simulink model "EST2"  (R2023b)
settings: Solver=FixedStepAuto  StartTime=0.0  StopTime=stopt  FixedStep=deltat  MaxStep=0.05  RelTol=1e-3
InitFcn:
  | clear all;
  | close all;
  | clc;
  | 
  | % add the data and script directories
  | addpath('data','scripts');
  | 
  | % load the constants (units)
  | constants;
  | 
  | % load the simulation parameters
  | preprocessing;
StopFcn:
  | postprocessing;
values from neighbouring files (symbols this model uses):
  aDemandTransport = aSupplyTransport    (= 0.97)    [preprocessing.m]
  aExtraction = 1- eta_extr    (= 0.1561)    [preprocessing.m]
  aSupplyTransport = 0.97    [preprocessing.m]
  bStorage = 0    [preprocessing.m]
  deltat = 5*unit("min")    [preprocessing.m]
  EStorageInitial = EStorageMax/2    (= 500000000000)    [preprocessing.m]
  EStorageMax = 1e12    (= 1000000000000)    [preprocessing.m]
  EStorageMin = EStorageMax/20    (= 50000000000)    [preprocessing.m]
  N_sphere = 35    [preprocessing.m]
  r_sph = 6.2    [preprocessing.m]
settings Model: Creator=joche  LastModifiedBy=20241276
settings DataIOCC: SaveFormat=Array  SaveOutput=off  ReturnWorkspaceOutputs=off
settings OptimizationCC: ReuseModelBlockBuffer=off
settings ModelReferenceCC: EnableRefExpFcnMdlSchedulingChecks=on

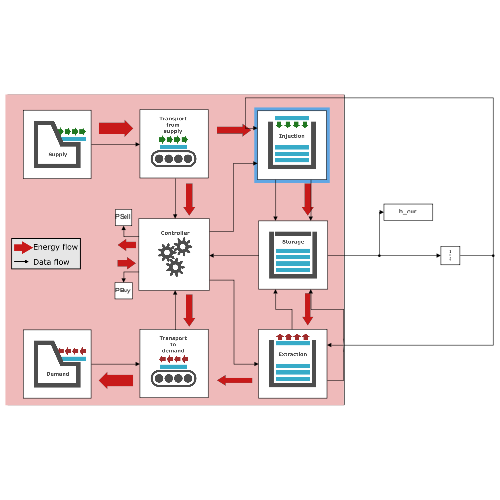
[thumbnail: Simulink's stored preview of the top-level diagram]
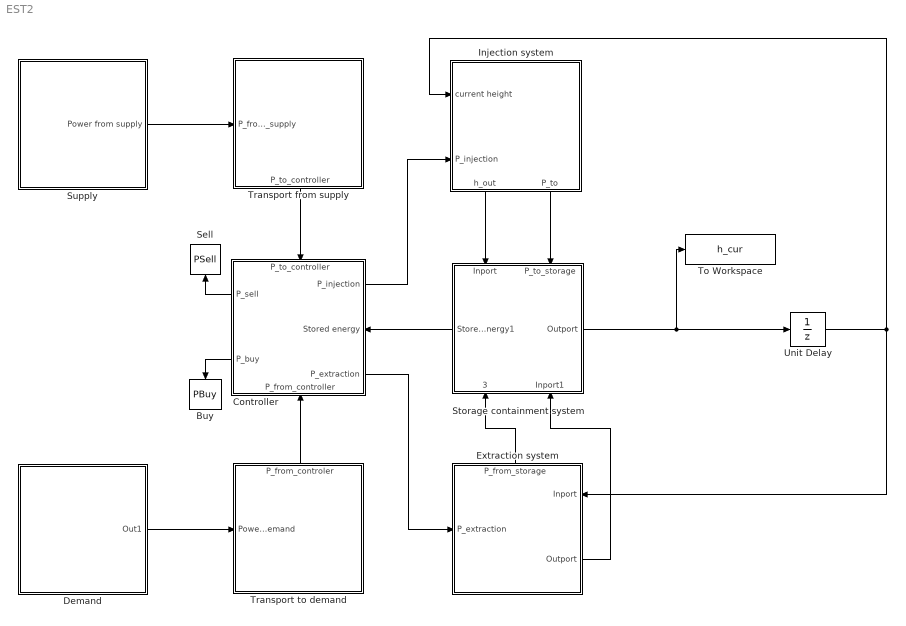
== system EST2 ==
  Buy : ToWorkspace  VariableName=PBuy  SampleTime=-1
  Controller : Subsystem
      settings: PortSchema="{\"entries\":[{\"content\":{\"sides\":[{\"content\":{\"connectorIds\":[\"Out3\",\"Out4\"]},\"type\":\"ConnectorPlacement.EquallySpacedRectSide\",\"uuid\":\"4daf33ce-c96a-4783-b5c4-228eed953e01\"},{\"content\":{\"connectorIds\":[\"Out1\",\"In3\",\"Out2\"],\"side\":\"RIGHT\"},\"type\":\"ConnectorPlacement.EquallySpacedRectSide\",\"uuid\":\"e9942e50-8467-4af8-b79b-80636cbc76e5\"},{\"content\":{\"connectorIds\":[\"In1\"],\"side\":\"TOP\"},\"type\":\"ConnectorPlacement.EquallySpacedRectSide\",\"uuid\":\"f315e931-d69b-4751-b712-f89c6c81baeb\"},{\"content\":{\"connectorIds\":[\"In2\"],\"side\":\"BOTTOM\"},\"type\":\"ConnectorPlacement.EquallySpacedRectSide\",\"uuid\":\"44715ee6-5cd5-4669-bcb9-5ed7c869bdb3\"}]},\"type\":\"ConnectorPlacement.EquallySpacedConnector\",\"uuid\":\"fff48899-944b-4064-b7d7-ecc12144fb48\"}],\"packageUris\":[\"http://schema.mathworks.com/mf0/Connector/R2020b\"],\"version\":\"1.0\"}"
      mask Display: image('$imagefile'); % Use "Edit Image" on toolstrip to change.
  Demand : Subsystem
      mask Display: image('$imagefile'); % Use "Edit Image" on toolstrip to change.
  Extraction system : Subsystem
      settings: PortSchema="{\"entries\":[{\"content\":{\"sides\":[{\"content\":{\"connectorIds\":[\"Out2\",\"In1\"]},\"type\":\"ConnectorPlacement.EquallySpacedRectSide\",\"uuid\":\"05c5933d-55fc-4e06-853f-fc26d42905f9\"},{\"content\":{\"connectorIds\":[\"In2\"],\"side\":\"RIGHT\"},\"type\":\"ConnectorPlacement.EquallySpacedRectSide\",\"uuid\":\"327426c5-31d5-498b-a2bd-83e49353408c\"},{\"content\":{\"side\":\"TOP\"},\"type\":\"ConnectorPlacement.EquallySpacedRectSide\",\"uuid\":\"55306cf3-a3de-4385-a5ae-b8600ecdd5a2\"},{\"content\":{\"connectorIds\":[\"Out1\"],\"side\":\"BOTTOM\"},\"type\":\"ConnectorPlacement.EquallySpacedRectSide\",\"uuid\":\"08fcc9c3-40d3-4ac6-b914-dfeef6039ffb\"}]},\"type\":\"ConnectorPlacement.EquallySpacedConnector\",\"uuid\":\"cb35d5ba-e8c6-462c-b7b2-fe8356d4b0a1\"}],\"packageUris\":[\"http://schema.mathworks.com/mf0/Connector/R2020b\"],\"version\":\"1.0\"}"
      mask Display: image('$imagefile'); % Use "Edit Image" on toolstrip to change.
  Injection system : Subsystem
      settings: PortSchema="{\"entries\":[{\"content\":{\"sides\":[{\"content\":{},\"type\":\"ConnectorPlacement.EquallySpacedRectSide\",\"uuid\":\"05c5933d-55fc-4e06-853f-fc26d42905f9\"},{\"content\":{\"connectorIds\":[\"In1\",\"In2\"],\"side\":\"RIGHT\"},\"type\":\"ConnectorPlacement.EquallySpacedRectSide\",\"uuid\":\"327426c5-31d5-498b-a2bd-83e49353408c\"},{\"content\":{\"connectorIds\":[\"Out1\",\"Out2\"],\"side\":\"TOP\"},\"type\":\"ConnectorPlacement.EquallySpacedRectSide\",\"uuid\":\"55306cf3-a3de-4385-a5ae-b8600ecdd5a2\"},{\"content\":{\"side\":\"BOTTOM\"},\"type\":\"ConnectorPlacement.EquallySpacedRectSide\",\"uuid\":\"08fcc9c3-40d3-4ac6-b914-dfeef6039ffb\"}]},\"type\":\"ConnectorPlacement.EquallySpacedConnector\",\"uuid\":\"cb35d5ba-e8c6-462c-b7b2-fe8356d4b0a1\"}],\"packageUris\":[\"http://schema.mathworks.com/mf0/Connector/R2020b\"],\"version\":\"1.0\"}"
      mask Display: image('$imagefile'); % Use "Edit Image" on toolstrip to change.
  Sell : ToWorkspace  VariableName=PSell  SampleTime=-1
  Storage containment system : Subsystem
      settings: PortSchema="{\"entries\":[{\"content\":{\"sides\":[{\"content\":{\"connectorIds\":[\"Out2\"]},\"type\":\"ConnectorPlacement.EquallySpacedRectSide\",\"uuid\":\"0ba48424-33b9-4934-970f-64fe5d8b070e\"},{\"content\":{\"connectorIds\":[\"Out1\"],\"side\":\"RIGHT\"},\"type\":\"ConnectorPlacement.EquallySpacedRectSide\",\"uuid\":\"9cde340f-8f39-4499-9a12-5e1623737660\"},{\"content\":{\"connectorIds\":[\"In1\",\"In2\"],\"side\":\"TOP\"},\"type\":\"ConnectorPlacement.EquallySpacedRectSide\",\"uuid\":\"2af8db04-7fd0-4902-8637-8dc00edb4598\"},{\"content\":{\"connectorIds\":[\"In3\",\"In4\"],\"side\":\"BOTTOM\"},\"type\":\"ConnectorPlacement.EquallySpacedRectSide\",\"uuid\":\"e21ea806-d777-41a3-a53f-556fae66854b\"}]},\"type\":\"ConnectorPlacement.EquallySpacedConnector\",\"uuid\":\"4e2ddb36-4db3-4ab4-858b-ebb8ccefeb1f\"}],\"packageUris\":[\"http://schema.mathworks.com/mf0/Connector/R2020b\"],\"version\":\"1.0\"}"
      mask Display: image('$imagefile'); % Use "Edit Image" on toolstrip to change.
  Supply : Subsystem
      mask Display: image('$imagefile'); % Use "Edit Image" on toolstrip to change.
  To Workspace : ToWorkspace  VariableName=h_cur  SaveFormat=Timeseries  SampleTime=-1
  Transport from supply : Subsystem
      settings: PortSchema="{\"entries\":[{\"content\":{\"sides\":[{\"content\":{\"connectorIds\":[\"In1\"]},\"type\":\"ConnectorPlacement.EquallySpacedRectSide\",\"uuid\":\"31329006-3d36-4d93-9c44-7503a515d397\"},{\"content\":{\"connectorIds\":[],\"side\":\"RIGHT\"},\"type\":\"ConnectorPlacement.EquallySpacedRectSide\",\"uuid\":\"aba139c7-f9b6-4881-a56b-a4cbbedacd88\"},{\"content\":{\"connectorIds\":[],\"side\":\"TOP\"},\"type\":\"ConnectorPlacement.EquallySpacedRectSide\",\"uuid\":\"e683eb73-7a35-4160-9c39-da83856a6278\"},{\"content\":{\"connectorIds\":[\"Out1\"],\"side\":\"BOTTOM\"},\"type\":\"ConnectorPlacement.EquallySpacedRectSide\",\"uuid\":\"1170dd18-447c-437f-9043-6812c2877331\"}]},\"type\":\"ConnectorPlacement.EquallySpacedConnector\",\"uuid\":\"804af608-1d70-444f-af69-e05f19bf98f3\"}],\"packageUris\":[\"http://schema.mathworks.com/mf0/Connector/R2020b\"],\"version\":\"1.0\"}"
      mask Display: image('$imagefile'); % Use "Edit Image" on toolstrip to change.
  Transport to demand : Subsystem
      settings: PortSchema="{\"entries\":[{\"content\":{\"sides\":[{\"content\":{\"connectorIds\":[\"In1\"]},\"type\":\"ConnectorPlacement.EquallySpacedRectSide\",\"uuid\":\"31329006-3d36-4d93-9c44-7503a515d397\"},{\"content\":{\"connectorIds\":[],\"side\":\"RIGHT\"},\"type\":\"ConnectorPlacement.EquallySpacedRectSide\",\"uuid\":\"aba139c7-f9b6-4881-a56b-a4cbbedacd88\"},{\"content\":{\"connectorIds\":[\"Out1\"],\"side\":\"TOP\"},\"type\":\"ConnectorPlacement.EquallySpacedRectSide\",\"uuid\":\"e683eb73-7a35-4160-9c39-da83856a6278\"},{\"content\":{\"connectorIds\":[],\"side\":\"BOTTOM\"},\"type\":\"ConnectorPlacement.EquallySpacedRectSide\",\"uuid\":\"c378138f-7233-4483-870c-40a69b3495ee\"}]},\"type\":\"ConnectorPlacement.EquallySpacedConnector\",\"uuid\":\"804af608-1d70-444f-af69-e05f19bf98f3\"}],\"packageUris\":[\"http://schema.mathworks.com/mf0/Connector/R2020b\"],\"version\":\"1.0\"}"
      mask Display: image('$imagefile'); % Use "Edit Image" on toolstrip to change.
  Unit Delay : UnitDelay  InitialCondition=r_sph  SampleTime=-1  HasFrameUpgradeWarning=on
  wires:
  Supply/1(Power from supply) -> Transport from supply/1(P_from_supply)
  Transport from supply/1(P_to_controller) -> Controller/1(P_to_controller)
  Transport to demand/1(P_from_controler) -> Controller/2(P_from_controller)
  Demand/1(Out1) -> Transport to demand/1(Power to demand)
  Controller/3(P_sell) -> Sell/1
  Controller/2(P_extraction) -> Extraction system/2(P_extraction)
  Injection system/1(P_to) -> Storage containment system/2(P_to_storage)
  Extraction system/1(P_from_storage) -> Storage containment system/3(P_from_storage)
  Storage containment system/2(Stored energy1) -> Controller/3(Stored energy)
  Controller/1(P_injection) -> Injection system/1(P_injection)
  Controller/4(P_buy) -> Buy/1
  Injection system/2(h_out) -> Storage containment system/1(Inport)
  Extraction system/2(Outport) -> Storage containment system/4(Inport1)
  Storage containment system/1(Outport) -> To Workspace/1, Unit Delay/1
  Unit Delay/1 -> Injection system/2(current height), Extraction system/1(Inport)

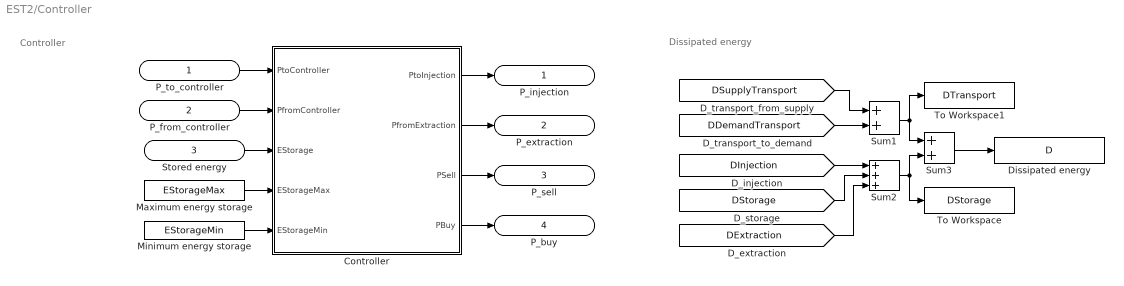
== system EST2/Controller ==
  note: Dissipated energy
  note: Controller
  P_to_controller : Inport
  P_from_controller : Inport  Port=2
  Stored energy : Inport  Port=3
  Controller : MATLAB Function  TreatAsAtomicUnit=on
  Dissipated energy : ToWorkspace  VariableName=D  SampleTime=-1
  Maximum energy storage : Constant  Value=EStorageMax
  Minimum energy storage : Constant  Value=EStorageMin
  Sum1 : Sum
  Sum2 : Sum  Inputs=+++
  Sum3 : Sum
  To Workspace : ToWorkspace  VariableName=DStorage  SampleTime=-1
  To Workspace1 : ToWorkspace  VariableName=DTransport  SampleTime=-1
  P_injection : Outport
  P_extraction : Outport  Port=2
  P_sell : Outport  Port=3
  P_buy : Outport  Port=4
  wires:
  P_from_controller/1 -> Controller/2(PfromController)
  Controller/2(PfromExtraction) -> P_extraction/1
  Controller/3(PSell) -> P_sell/1
  Controller/4(PBuy) -> P_buy/1
  Minimum energy storage/1 -> Controller/5(EStorageMin)
  Maximum energy storage/1 -> Controller/4(EStorageMax)
  P_to_controller/1 -> Controller/1(PtoController)
  Controller/1(PtoInjection) -> P_injection/1
  Stored energy/1 -> Controller/3(EStorage)
  [DDemandTransport] -> Sum1/2
  [DSupplyTransport] -> Sum1/1
  [DInjection] -> Sum2/1
  [DStorage] -> Sum2/2
  [DExtraction] -> Sum2/3
  Sum2/1 -> To Workspace/1, Sum3/2
  Sum1/1 -> To Workspace1/1, Sum3/1
  Sum3/1 -> Dissipated energy/1

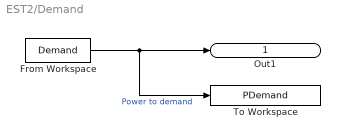
== system EST2/Demand ==
  From Workspace : FromWorkspace  VariableName=Demand  OutputAfterFinalValue=Setting to zero
  To Workspace : ToWorkspace  VariableName=PDemand  SampleTime=-1
  Out1 : Outport
  wires:
  From Workspace/1 -> To Workspace/1, Out1/1  "Power to demand"

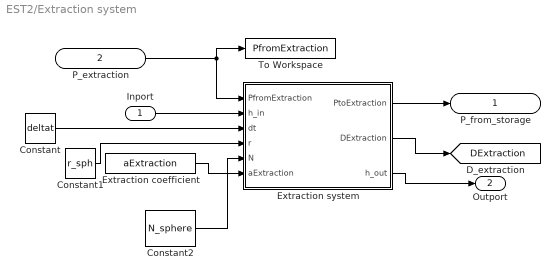
== system EST2/Extraction system ==
  Inport : Inport
  P_extraction : Inport  Port=2
  Constant : Constant  Value=deltat
  Constant1 : Constant  Value=r_sph
  Constant2 : Constant  Value=N_sphere
  Extraction coefficient : Constant  Value=aExtraction
  Extraction system : MATLAB Function  TreatAsAtomicUnit=on
  To Workspace : ToWorkspace  VariableName=PfromExtraction  SampleTime=-1
  P_from_storage : Outport
  Outport : Outport  Port=2
  tag scope: DExtraction=global
  wires:
  P_extraction/1 -> Extraction system/1(PfromExtraction), To Workspace/1
  Extraction system/1(PtoExtraction) -> P_from_storage/1
  Extraction coefficient/1 -> Extraction system/6(aExtraction)
  Extraction system/2(DExtraction) -> [DExtraction]
  Inport/1 -> Extraction system/2(h_in)
  Extraction system/3(h_out) -> Outport/1
  Constant/1 -> Extraction system/3(dt)
  Constant2/1 -> Extraction system/5(N)
  Constant1/1 -> Extraction system/4(r)

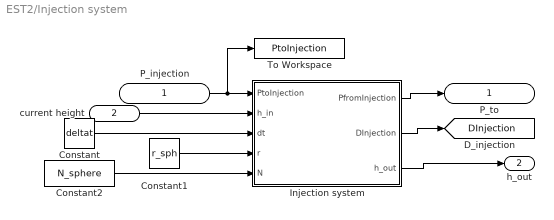
== system EST2/Injection system ==
  P_injection : Inport
  current height : Inport  Port=2
  Constant : Constant  Value=deltat
  Constant1 : Constant  Value=r_sph
  Constant2 : Constant  Value=N_sphere
  Injection system : MATLAB Function  TreatAsAtomicUnit=on
  To Workspace : ToWorkspace  VariableName=PtoInjection  SampleTime=-1
  P_to : Outport
  h_out : Outport  Port=2
  tag scope: DInjection=global
  wires:
  P_injection/1 -> To Workspace/1, Injection system/1(PtoInjection)
  Injection system/1(PfromInjection) -> P_to/1
  Injection system/2(DInjection) -> [DInjection]
  Injection system/3(h_out) -> h_out/1
  current height/1 -> Injection system/2(h_in)
  Constant/1 -> Injection system/3(dt)
  Constant2/1 -> Injection system/5(N)
  Constant1/1 -> Injection system/4(r)

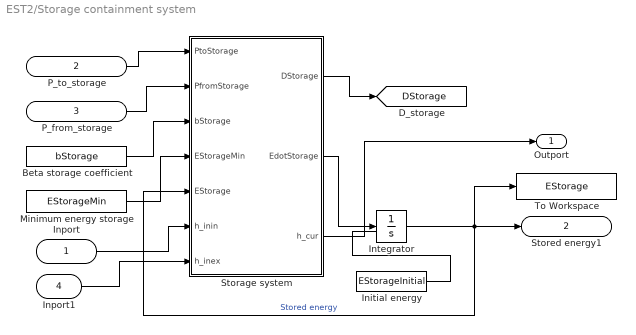
== system EST2/Storage containment system ==
  Inport : Inport
  P_to_storage : Inport  Port=2
  P_from_storage : Inport  Port=3
  Inport1 : Inport  Port=4
  Beta storage coefficient : Constant  Value=bStorage
  Initial energy : Constant  Value=EStorageInitial
  Integrator : Integrator
  Minimum energy storage : Constant  Value=EStorageMin
  Storage system : MATLAB Function  TreatAsAtomicUnit=on
  To Workspace : ToWorkspace  VariableName=EStorage  SampleTime=-1
  Outport : Outport
  Stored energy1 : Outport  Port=2
  tag scope: DStorage=global
  wires:
  P_from_storage/1 -> Storage system/2(PfromStorage)
  P_to_storage/1 -> Storage system/1(PtoStorage)
  Initial energy/1 -> ?
  Integrator/1 -> To Workspace/1, Storage system/5(EStorage), Stored energy1/1  "Stored energy"
  Storage system/1(DStorage) -> [DStorage]
  Beta storage coefficient/1 -> Storage system/3(bStorage)
  Storage system/2(EdotStorage) -> Integrator/1
  Minimum energy storage/1 -> Storage system/4(EStorageMin)
  Inport/1 -> Storage system/6(h_inin)
  Storage system/3(h_cur) -> Outport/1
  Inport1/1 -> Storage system/7(h_inex)

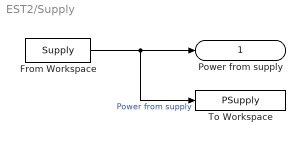
== system EST2/Supply ==
  From Workspace : FromWorkspace  VariableName=Supply  OutputAfterFinalValue=Setting to zero
  To Workspace : ToWorkspace  VariableName=PSupply  SampleTime=-1
  Power from supply : Outport
  wires:
  From Workspace/1 -> To Workspace/1, Power from supply/1  "Power from supply"

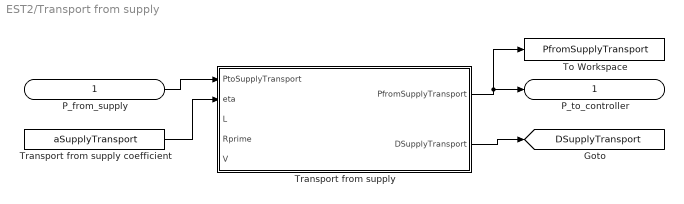
== system EST2/Transport from supply ==
  P_from_supply : Inport
  To Workspace : ToWorkspace  VariableName=PfromSupplyTransport  SampleTime=-1
  Transport from supply : MATLAB Function  TreatAsAtomicUnit=on
  Transport from supply coefficient : Constant  Value=aSupplyTransport
  P_to_controller : Outport
  tag scope: DSupplyTransport=global
  wires:
  Transport from supply coefficient/1 -> Transport from supply/2(eta)
  P_from_supply/1 -> Transport from supply/1(PtoSupplyTransport)
  Transport from supply/1(PfromSupplyTransport) -> To Workspace/1, P_to_controller/1
  Transport from supply/2(DSupplyTransport) -> [DSupplyTransport]

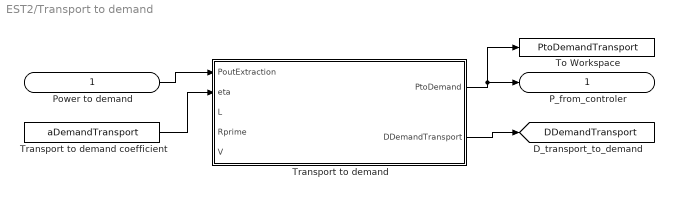
== system EST2/Transport to demand ==
  Power to demand : Inport
  To Workspace : ToWorkspace  VariableName=PtoDemandTransport  SampleTime=-1
  Transport to demand : MATLAB Function  TreatAsAtomicUnit=on
  Transport to demand coefficient : Constant  Value=aDemandTransport
  P_from_controler : Outport
  tag scope: DDemandTransport=global
  wires:
  Transport to demand coefficient/1 -> Transport to demand/2(eta)
  Power to demand/1 -> Transport to demand/1(PoutExtraction)
  Transport to demand/1(PtoDemand) -> To Workspace/1, P_from_controler/1
  Transport to demand/2(DDemandTransport) -> [DDemandTransport]

== matlab function EST2/Injection system/Injection system ==
  data: PtoInjection input; h_in input; PfromInjection output; dt input; DInjection output; h_out output; r input; N input

function [PfromInjection, DInjection, h_out] = computeInjectionSimulink(PtoInjection, h_in, dt,r,N)
% Calculates stored power, loss, and new tank height from pump input

 % Physical constants
    rho = 1000;          % Water density [kg/m^3]
    g = 9.81;            % Gravity [m/s^2]
    r_sph_small  = r;
    N_small = N;
    depth = 100;
% Pump and converter efficiency
eta_converter = 0.97;
eta_pump = 0.80;
eta_inj = eta_converter * eta_pump;

H_eff = depth - h_in;

% Pumped mass (kg): m = (eta * P * dt) / (g * H_eff)
m_pumped = eta_inj * PtoInjection * dt / (g * H_eff);
V_pumped = m_pumped / rho;   % [m^3]

% Total tank cross-sectional volume at this height
% For inverse spherical cap: use differential volume approximation
% Instead, solve new height numerically (simplified here)

% Add volume to tank (assuming uniform distribution)
V_total = (pi * h_in^2 * (3*r_sph_small - h_in)) / 3 + V_pumped / N_small;


% Solve for new height from volume
% Use Newton-Raphson or brute-force (we’ll use simple loop approx here)
h_out = h_in;
for i = 1:10
    V_guess = (pi * h_out^2 * (3*r_sph_small - h_out)) / 3;
    error = V_guess - V_total;
    dVdh = pi * h_out * (3*r_sph_small - h_out); % derivative dV/dh
    h_out = h_out - error / dVdh;
    h_out = max(0, min(h_out, 2 * r_sph_small));
end

% Potential energy added
E_added = m_pumped * g * H_eff;
PfromInjection = E_added / dt;
DInjection = PtoInjection - PfromInjection;
end

== matlab function EST2/Transport from supply/Transport from supply ==
  data: PtoSupplyTransport input; PfromSupplyTransport output; eta input; DSupplyTransport output; L input; Rprime input; V input
function [PfromSupplyTransport, DSupplyTransport] = supplyTransport(PtoSupplyTransport, eta, L, Rprime, V)
    % supplyTransport: Calculates power delivered after transport, considering losses
    % PtoSupplyTransport : Power intended to be transported [W]
    % eta                : Transformer efficiency
    % L                  : Cable length [km]
    % Rprime             : Resistance per unit length [Ohm/km]
    % V                  : Transmission voltage [V]
    % Returns:
    % PfromSupplyTransport : Power delivered after transport [W]
    % DSupplyTransport     : Total power losses during transport [W]

    % Calculate power after transport using the formula
    PfromSupplyTransport = eta^2 * PtoSupplyTransport - eta^3 * L * Rprime * (PtoSupplyTransport^2) / (V^2);

    % Calculate the total losses
    DSupplyTransport = PtoSupplyTransport - PfromSupplyTransport;
end

== matlab function EST2/Controller/Controller ==
  data: PtoInjection output; PfromExtraction output; PSell output; PBuy output; PtoController input; PfromController input; EStorage input; EStorageMax input; EStorageMin input
function [PtoInjection, PfromExtraction, PSell, PBuy] = controller(PtoController, PfromController, EStorage, EStorageMax, EStorageMin)
    
    %% Power surplus or deficit

    deltaP = PtoController - PfromController;

    % Power surplus
    if deltaP >= 0

        %% Storage injection

        % Storage system is not full
        if EStorage < EStorageMax 

            PtoInjection = deltaP;

        % Storage system is full
        else
            PtoInjection = 0;
        end

        %% Storage extraction

        PfromExtraction = 0;

        %% Load-balancing
        PSell   = deltaP - PtoInjection;
        PBuy    = 0;

    % Power deficit
    else

        %% Storage injection

        PtoInjection = 0;

        %% Storage extraction

        % Storage system is not empty
        if EStorage > EStorageMin

            PfromExtraction = -deltaP;

        % Storage system is empty
        else
            PfromExtraction = 0;
        end

        %% Load-balancing

        PSell = 0;
        PBuy  = -deltaP - PfromExtraction;
    end

== matlab function EST2/Extraction system/Extraction system ==
  data: PfromExtraction input; h_in input; dt input; r input; N input; PtoExtraction output; aExtraction input; DExtraction output; h_out output
function [PtoExtraction, DExtraction, h_out] = extraction(PfromExtraction, h_in, dt, r, N, aExtraction)
% Computes electrical power output and updated tank height from water inflow (turbine extraction)

    % Physical constants
    rho = 1000;      % Water density [kg/m^3]
    g = 9.81;        % Gravitational acceleration [m/s^2]
    depth = 100;     % Height of upper reservoir relative to seabed [m]

    % Tank geometry
    r_sph = r;
    N_sphere = N;

    % Turbine efficiency
    eta_extr = aExtraction;

    % Effective head: height difference from centroid of water to upper reservoir
    h = max(0, min(h_in, 2 * r_sph));
    H_eff = depth - h;

    % Hydraulic energy input
    E_hydraulic = PfromExtraction * dt;

    % Mass of water needed to extract this energy
    m_water = E_hydraulic / (g * H_eff);
    V_water = m_water / rho;
    V_water_per_tank = V_water / N_sphere;

    % Initial volume
    V_initial = (pi * h^2 * (3 * r_sph - h)) / 3;
    V_total = V_initial + V_water_per_tank;

    % Solve for new height using Newton-Raphson
    h_out = h;
    for i = 1:10
        V_guess = (pi * h_out^2 * (3 * r_sph - h_out)) / 3;
        error = V_guess - V_total;
        dVdh = pi * h_out * (3 * r_sph - h_out);
        h_out = h_out - error / dVdh;
        h_out = max(0, min(h_out, 2 * r_sph));
    end

    % Electrical output
    E_electric = E_hydraulic * eta_extr;
    PtoExtraction = E_electric / dt;

    % Losses
    DExtraction = PfromExtraction - PtoExtraction;
end

== matlab function EST2/Storage containment system/Storage system ==
  settings: updateMethod=DISCRETE
  data: DStorage output; EdotStorage output; PtoStorage input; PfromStorage input; bStorage input; EStorageMin input; EStorage input; h_inin input; h_cur output; h_inex input
function [DStorage, EdotStorage, h_cur] = Storage(PtoStorage, PfromStorage, bStorage, EStorageMin, EStorage, h_inin, h_inex)
% Storage : Models storage self-discharge and energy rate of change
% PtoStorage   : Power input to storage [W]
% PfromStorage : Power output from storage [W]
% bStorage     : Storage dissipation coefficient [1/s]
% EStorageMin  : Minimum storage energy [J]
% EStorage     : Current storage energy [J]
% h_inin, h_inex : Heights from injection and extraction

% Persistent variables to track previous states
persistent h_prev_inin h_prev_inex h_cur_prev

% Initialize persistent variables on first run
if isempty(h_prev_inin)
    h_prev_inin = h_inin;
    h_prev_inex = h_inex;
    h_cur_prev = min([h_inin, h_inex]); % Default initialization
end

% Calculate changes
delta_inin = h_inin - h_prev_inin;
delta_inex = h_inex - h_prev_inex;

% Determine h_cur based on changes
if delta_inin ~= 0 && delta_inex ~= 0
    h_cur = h_cur_prev + delta_inin + delta_inex;
elseif delta_inin ~= 0
    h_cur = h_inin;
elseif delta_inex ~= 0
    h_cur = h_inex;
else
    h_cur = h_cur_prev; % No change
end

% Update persistent values
h_prev_inin = h_inin;
h_prev_inex = h_inex;
h_cur_prev = h_cur;

% Storage power loss and energy change
DStorage = bStorage * (EStorage - EStorageMin);
EdotStorage = PtoStorage - PfromStorage - DStorage;
end

== matlab function EST2/Transport to demand/Transport to demand ==
  data: PoutExtraction input; PtoDemand output; eta input; DDemandTransport output; L input; Rprime input; V input
function [PtoDemand, DDemandTransport] = demandTransport(PoutExtraction, eta, L, Rprime, V)
% demandTransport : Calculates delivered power and losses for transport to demand
% PoutExtraction      : Power output from extraction block [W]
% eta                 : Transformer efficiency (0 < eta <= 1)
% L                   : Cable length [km]
% Rprime              : Cable resistance per unit length [Ohm/km]
% V                   : Transmission voltage [V]
% Returns:
% PtoDemand           : Power delivered to demand [W]
% DDemandTransport    : Total power losses during transport [W]

PtoDemand = eta^2 * PoutExtraction - eta^3 * L * Rprime * (PoutExtraction^2) / (V^2);
DDemandTransport = PoutExtraction - PtoDemand;
end
